simulink model "nn_and"  (R2018b)
settings: Solver=VariableStepAuto  StartTime=0.0  StopTime=10.0  RelTol=1e-3
libraries: neural x4
settings Model: Creator=Mihail  LastModifiedBy=Mihail

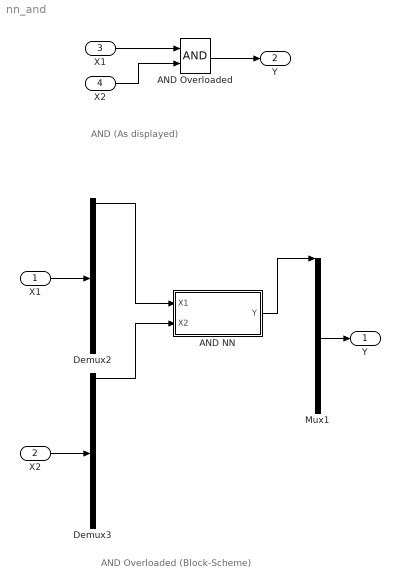
== system nn_and ==
  note: AND Overloaded
      | (Block-Scheme)
  note: AND (As displayed)
  "X1 " : Inport
  "X2 " : Inport  Port=2
  X1 : Inport  Port=3
  X2 : Inport  Port=4
  AND NN : Subsystem
  AND Overloaded : Logic  AllPortsSameDT=off  OutDataTypeStr=boolean
  Demux2 : Demux  Outputs=32
  Demux3 : Demux  Outputs=32
  Mux1 : Mux  Inputs=32
  "Y " : Outport
  Y : Outport  Port=2
  wires:
  AND NN/1(Y) -> Mux1/1
  "X2 "/1 -> Demux3/1
  Demux2/2 -> AND NN/1(X1)
  "X1 "/1 -> Demux2/1
  Demux3/2 -> AND NN/2(X2)
  Mux1/1 -> "Y "/1
  X1/1 -> AND Overloaded/1
  X2/1 -> AND Overloaded/2
  AND Overloaded/1 -> Y/1

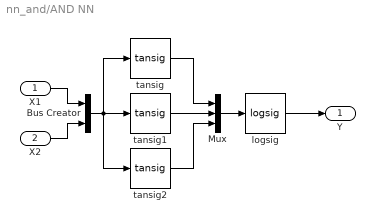
== system nn_and/AND NN ==
  X1 : Inport
  X2 : Inport  Port=2
  Bus Creator : BusCreator  Inputs=2
  Mux : Mux  Inputs=3
  logsig : neural/Transfer Functions/logsig
  tansig : neural/Transfer Functions/tansig
  tansig1 : neural/Transfer Functions/tansig
  tansig2 : neural/Transfer Functions/tansig
  Y : Outport
  wires:
  tansig2/1 -> Mux/3
  tansig1/1 -> Mux/2
  tansig/1 -> Mux/1
  Mux/1 -> logsig/1
  logsig/1 -> Y/1
  X1/1 -> Bus Creator/1
  X2/1 -> Bus Creator/2
  Bus Creator/1 -> tansig/1, tansig2/1, tansig1/1
